simulink model "EKF_onlyparameters"  (R2020b)
settings: Solver=VariableStepAuto  StartTime=0.0  StopTime=time  RelTol=1e-3
values from neighbouring files (symbols this model uses):
  Ath = 0.5    [main.m]
  b = sym('b','real')    [Oss_par.m]    (also in main.m = 0.2)
  gravity = sym('gravity','real')    [Oss_par.m]    (also in main.m = 9.81)
  I = sym('I','real')    [Oss_par.m]    (also in main.m = 235.2)
  K = sym('K','real')    [Oss_par.m]    (also in main.m = 40.248)
  L = sym('L','real')    [Oss_par.m]    (also in dir_der.m = h * f; main.m = 2.1)
  m = sym('m','real')    [Oss_par.m]    (also in main.m = 160)
  R = sym('R','real')    [Oss_par.m]    (also in main.m = 0.6)
  selector = select(1)    [main.m]    (also in select.m = input('? '))
  wth = 0.2    [main.m]
settings Model: Creator=Tommaso  LastModifiedBy=Tommaso
settings DataIOCC: ReturnWorkspaceOutputs=off

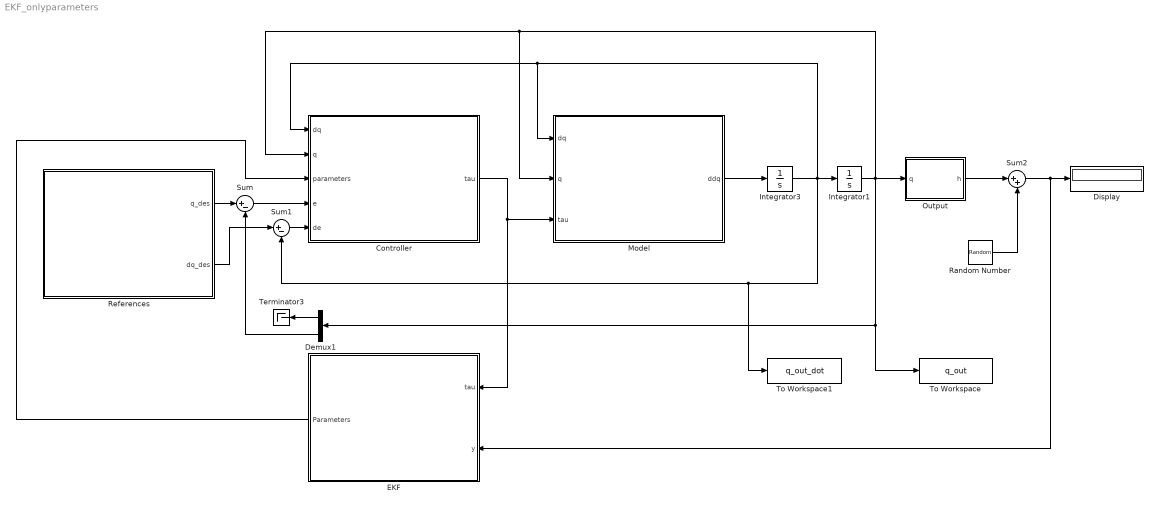
== system EKF_onlyparameters ==
  Controller : MATLAB Function  TreatAsAtomicUnit=on
  Demux1 : Demux  Outputs=2
  Display : Display
  EKF : Subsystem
  Integrator1 : Integrator  InitialCondition=[0; pi/12]
  Integrator3 : Integrator  InitialCondition=[0; 0]
  Model : MATLAB Function  TreatAsAtomicUnit=on
  Output : MATLAB Function  TreatAsAtomicUnit=on
  Random Number : RandomNumber  Variance=0.000003  Seed=24  SampleTime=0.1
  References : Subsystem
  Sum : Sum  Inputs=|+-
  Sum1 : Sum  Inputs=|+-
  Sum2 : Sum  Inputs=|++
  Terminator3 : Terminator
  To Workspace : ToWorkspace  VariableName=q_out  SaveFormat=Timeseries  SampleTime=-1
  To Workspace1 : ToWorkspace  VariableName=q_out_dot  SaveFormat=Timeseries  SampleTime=-1
  wires:
  Demux1/2 -> Sum/2
  Controller/1(tau) -> Model/3(tau), EKF/1(tau)
  Output/1(h) -> Sum2/1
  Random Number/1 -> Sum2/2
  Demux1/1 -> Terminator3/1
  Sum1/1 -> Controller/5(de)
  Model/1(ddq) -> Integrator3/1
  Sum/1 -> Controller/4(e)
  Integrator3/1 -> To Workspace1/1, Sum1/2, Integrator1/1, Model/1(dq), Controller/1(dq)
  Integrator1/1 -> To Workspace/1, Demux1/1, Output/1(q), Model/2(q), Controller/2(q)
  Sum2/1 -> EKF/2(y), Display/1
  References/1(q_des) -> Sum/1
  References/2(dq_des) -> Sum1/1
  EKF/1(Parameters) -> Controller/3(parameters)

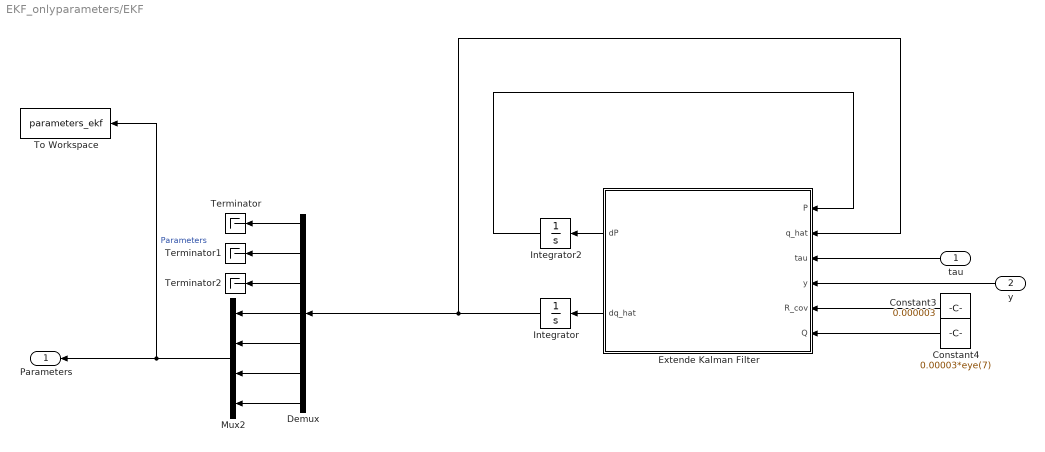
== system EKF_onlyparameters/EKF ==
  tau : Inport
  y : Inport  Port=2
  Constant3 : Constant  Value=0.000003
  Constant4 : Constant  Value=0.00003*eye(7)
  Demux : Demux  Outputs=7
  Extende Kalman Filter : MATLAB Function  TreatAsAtomicUnit=on
  Integrator : Integrator  InitialCondition=[0; 0; 0; 158; 238; 0.15; 41]
  Integrator2 : Integrator  InitialCondition=0*eye(7)
  Mux2 : Mux
  Terminator : Terminator
  Terminator1 : Terminator
  Terminator2 : Terminator
  To Workspace : ToWorkspace  VariableName=parameters_ekf  SaveFormat=Timeseries  SampleTime=-1
  Parameters : Outport
  wires:
  Mux2/1 -> To Workspace/1, Parameters/1  "Parameters"
  Demux/4 -> Mux2/1
  Demux/5 -> Mux2/2
  Demux/6 -> Mux2/3
  Demux/3 -> Terminator2/1
  Demux/7 -> Mux2/4
  Demux/2 -> Terminator1/1
  Integrator/1 -> Extende Kalman Filter/2(q_hat), Demux/1
  Demux/1 -> Terminator/1
  Constant4/1 -> Extende Kalman Filter/6(Q)
  Extende Kalman Filter/2(dq_hat) -> Integrator/1
  Constant3/1 -> Extende Kalman Filter/5(R_cov)
  Extende Kalman Filter/1(dP) -> Integrator2/1
  Integrator2/1 -> Extende Kalman Filter/1(P)
  tau/1 -> Extende Kalman Filter/3(tau)
  y/1 -> Extende Kalman Filter/4(y)

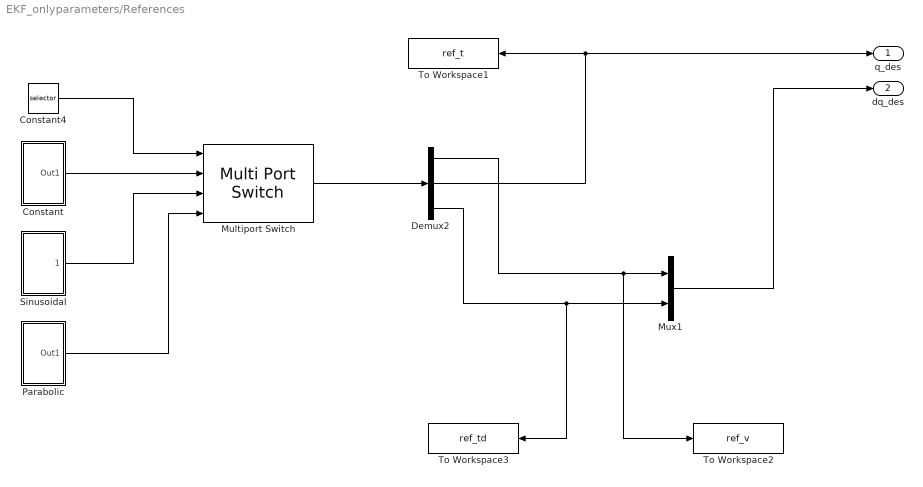
== system EKF_onlyparameters/References ==
  Constant : Subsystem
  Constant4 : Constant  Value=selector
  Demux2 : Demux  Outputs=3
  Multiport Switch : MultiPortSwitch
  Mux1 : Mux  Inputs=2
  Parabolic : Subsystem
  Sinusoidal : Subsystem
  To Workspace1 : ToWorkspace  VariableName=ref_t  SaveFormat=Timeseries  SampleTime=-1
  To Workspace2 : ToWorkspace  VariableName=ref_v  SaveFormat=Timeseries  SampleTime=-1
  To Workspace3 : ToWorkspace  VariableName=ref_td  SaveFormat=Timeseries  SampleTime=-1
  q_des : Outport
  dq_des : Outport  Port=2
  wires:
  Mux1/1 -> dq_des/1
  Demux2/2 -> q_des/1, To Workspace1/1
  Multiport Switch/1 -> Demux2/1
  Sinusoidal/1(Outport) -> Multiport Switch/3
  Constant4/1 -> Multiport Switch/1
  Parabolic/1(Out1) -> Multiport Switch/4
  Demux2/1 -> To Workspace2/1, Mux1/1
  Constant/1(Out1) -> Multiport Switch/2
  Demux2/3 -> To Workspace3/1, Mux1/2

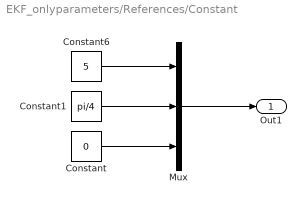
== system EKF_onlyparameters/References/Constant ==
  Constant : Constant  Value=0
  Constant1 : Constant  Value=pi/4
  Constant6 : Constant  Value=5
  Mux : Mux  Inputs=3
  Out1 : Outport
  wires:
  Constant1/1 -> Mux/2
  Constant/1 -> Mux/3
  Mux/1 -> Out1/1
  Constant6/1 -> Mux/1

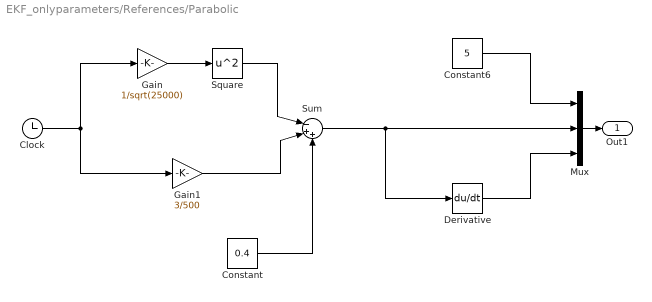
== system EKF_onlyparameters/References/Parabolic ==
  Clock : Clock
  Constant : Constant  Value=0.4
  Constant6 : Constant  Value=5
  Derivative : Derivative
  Gain : Gain  Gain=1/sqrt(25000)
  Gain1 : Gain  Gain=3/500
  Mux : Mux  Inputs=3
  Square : Math  Operator=square  SaturateOnIntegerOverflow=on
  Sum : Sum  Inputs=|-++
  Out1 : Outport
  wires:
  Mux/1 -> Out1/1
  Gain/1 -> Square/1
  Derivative/1 -> Mux/3
  Square/1 -> Sum/1
  Sum/1 -> Mux/2, Derivative/1
  Gain1/1 -> Sum/2
  Clock/1 -> Gain1/1, Gain/1
  Constant6/1 -> Mux/1
  Constant/1 -> Sum/3

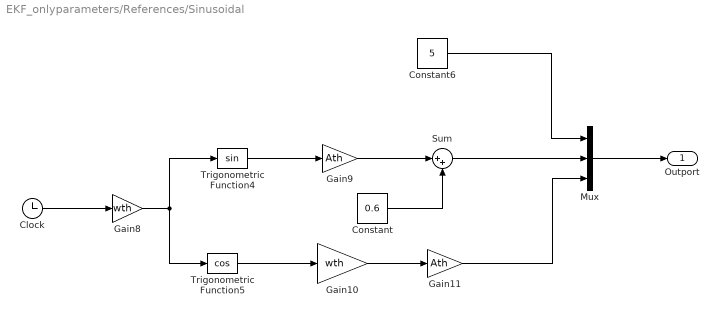
== system EKF_onlyparameters/References/Sinusoidal ==
  Clock : Clock
  Constant : Constant  Value=0.6
  Constant6 : Constant  Value=5
  Gain10 : Gain  Gain=wth
  Gain11 : Gain  Gain=Ath
  Gain8 : Gain  Gain=wth
  Gain9 : Gain  Gain=Ath
  Mux : Mux  Inputs=3
  Sum : Sum  Inputs=|++
  Trigonometric Function4 : Trigonometry
  Trigonometric Function5 : Trigonometry  Operator=cos
  Outport : Outport
  wires:
  Gain11/1 -> Mux/3
  Trigonometric Function5/1 -> Gain10/1
  Gain10/1 -> Gain11/1
  Gain8/1 -> Trigonometric Function4/1, Trigonometric Function5/1
  Constant/1 -> Sum/2
  Clock/1 -> Gain8/1
  Gain9/1 -> Sum/1
  Mux/1 -> Outport/1
  Trigonometric Function4/1 -> Gain9/1
  Sum/1 -> Mux/2
  Constant6/1 -> Mux/1

== matlab function EKF_onlyparameters/Output ==
  data: q input; h output; L parameter
function h = output(q, L)

% Output
h = L*sin(q(2));

== matlab function EKF_onlyparameters/Model ==
  data: m parameter; R parameter; gravity parameter; L parameter; dq input size=[2;1]; K parameter; b parameter; I parameter; q input size=[2;1]; tau input; ddq output
function ddq = model(m, R, gravity, L, dq, K, b, I, q, tau)

% Configuration variables
theta = q(2);
x_dot = dq(1);

% Inertial matrix (2x2)
M = [m*R 0; 0 I];

% Damping matrix (2x2)
C = [(R/2)*K*(1+sin(theta))*x_dot 0; -(L/4)*K*(1+sin(theta))*x_dot*sin(theta) b];

% Potential vector (2x1)
G = [0; m*gravity*(L/2)*cos(theta)];

% Dynamic equation
ddq = M^(-1)*(tau - C*dq - G);

== matlab function EKF_onlyparameters/Controller ==
  data: dq input; q input; parameters input; tau output; R parameter; gravity parameter; L parameter; e input; de input
function tau = controller(dq, q, parameters, R, gravity, L, e, de)

% Configurations variables
theta = q(2);
x_dot = dq(1);
m = parameters(1);
I = parameters(2);
b = parameters(3);
K = parameters(4);

% Gains
Kv = 200*eye(2);
Kp = 800*eye(2);

% Inertial matrix (2x2)
M = [m*R 0; 0 I];

% Damping matrix (2x2)
C = [(R/2)*K*(1+sin(theta))*x_dot 0; -(L/4)*K*(1+sin(theta))*x_dot*sin(theta) b];

% Potential vector (2x1)
G = [0; m*gravity*(L/2)*cos(theta)];

% Errors
E = [0; e];
dE = de;

% Control output (2x1)
tau = (Kv*dE + Kp*E) + C*dq + G;

% tau moltiplicato per M, Kv = 20 e Kp = 80

== matlab function EKF_onlyparameters/EKF/Extende Kalman Filter ==
  data: dP output; P input; dq_hat output; q_hat input size=[7;1]; L parameter; gravity parameter; tau input; y input; R parameter; R_cov input; Q input
function [dP, dq_hat] = EKF(P, q_hat, L, gravity, tau, y, R, R_cov, Q)

% Configuration variables
x_dot = q_hat(1);
theta = q_hat(2);
theta_dot = q_hat(3);
m = q_hat(4);
I = q_hat(5);
b = q_hat(6);
K = q_hat(7);

% Input vector (7x1)
tau_v = [tau(1); 0; tau(2); 0; 0; 0; 0];

% Drift field (7x1)
f = [-(1/m)*(K/2)*(1 + sin(theta))*x_dot^2; theta_dot; (1/I)*(((L/4)*(x_dot^2)*K*(1 + sin(theta))*sin(theta)) - b*theta_dot - m*gravity*(L/2)*cos(theta)); 0; 0; 0; 0];

% Control field (7x1)
g = [1/(m*R); 0; 1/I; 0; 0; 0; 0];

% Predicted output
h = L*sin(theta);

% Output jacobian (1x7)
H = [0, L*cos(theta), 0, 0, 0, 0, 0];

% System jacobian (7x7)
F = [                -(K*x_dot*(sin(theta) + 1))/m,                                                                                        -(K*x_dot^2*cos(theta))/(2*m),    0, (K*x_dot^2*(sin(theta) + 1))/(2*m^2),                                                                                            0,            0,             -(x_dot^2*(sin(theta) + 1))/(2*m)
                                                0,                                                                                                                    0,    1,                                    0,                                                                                            0,            0,                                             0
    (K*L*x_dot*sin(theta)*(sin(theta) + 1))/(2*I), ((L*gravity*m*sin(theta))/2 + (K*L*x_dot^2*cos(theta)*sin(theta))/4 + (K*L*x_dot^2*cos(theta)*(sin(theta) + 1))/4)/I, -b/I,        -(L*gravity*cos(theta))/(2*I), (b*theta_dot + (L*gravity*m*cos(theta))/2 - (K*L*x_dot^2*sin(theta)*(sin(theta) + 1))/4)/I^2, -theta_dot/I, (L*x_dot^2*sin(theta)*(sin(theta) + 1))/(4*I)
                                                0,                                                                                                                    0,    0,                                    0,                                                                                            0,            0,                                             0
                                                0,                                                                                                                    0,    0,                                    0,                                                                                            0,            0,                                             0
                                                0,                                                                                                                    0,    0,                                    0,                                                                                            0,            0,                                             0
                                                0,                                                                                                                    0,    0,                                    0,                                                                                            0,            0,                                             0];

% Kalman gain (7x1)
Kg = P*H'*inv(R_cov);

% Covariance error (7x7)
dP = F*P + P*F' - Kg*H*P + Q;

% System (7x1)
dq_hat = f + g.*tau_v + Kg*(y - h);
